simulink model "simulate_H_inf"  (R2013b)
settings: Solver=FixedStepDiscrete  StartTime=0.0  StopTime=100  FixedStep=T_s  RelTol=1e-3
values from neighbouring files (symbols this model uses):
  A = [0 0                                                1 0 ... (first row only)    [H_inf_state_feedback.m]    (also in Hinf_discrete_state_feedback_control (Dogan Onur ARISOY's conflicted copy 2017-02-06).m = a; Hinf_discrete_state_feedback_control.m = a; Hinf_discrete_state_feedback_control_ceyrek_tasit.m = a; bina_sistem.m = [zeros(4,4)         eye(4))
  B1 = [0;0;0;k2/m2]    [H_inf_state_feedback.m]    (also in Hinf_discrete_state_feedback_control (Dogan Onur ARISOY's conflicted copy 2017-02-06).m = b(:,1:size(Bc1,2)); Hinf_discrete_state_feedback_control.m = b(:,1:size(Bc1,2)); Hinf_discrete_state_feedback_control_ceyrek_tasit.m = b(:,1:size(Bc1,2)); bina_sistem.m = zeros(8,2))
  C = c(1:size(Cc1,1),:)    [Hinf_discrete_state_feedback_control (Dogan Onur ARISOY's conflicted copy 2017-02-06).m]    (also in Hinf_discrete_state_feedback_control.m; Hinf_discrete_state_feedback_control_ceyrek_tasit.m; bina_sistem.m = [c1+c2          -c2              0             0; dis_state_space.m)
  K = W*inv(X)    [H_inf_state_feedback.m]    (also in Hinf_discrete_state_feedback_control (Dogan Onur ARISOY's conflicted copy 2017-02-06).m = Y*Q^-1; Hinf_discrete_state_feedback_control.m = [k1 -k1;-k1 k1+k2]; Hinf_discrete_state_feedback_control_ceyrek_tasit.m = Y*Q^-1; LMI_state.m)
  T_s = 1e-6    (= 1e-06)    [Hinf_discrete_state_feedback_control (Dogan Onur ARISOY's conflicted copy 2017-02-06).m]    (also in Hinf_discrete_state_feedback_control.m = 0.0001; Hinf_discrete_state_feedback_control_ceyrek_tasit.m = 0.01; bench__lmi_state_hinf.m = 0.01; bina__lmi_state_hinf.m = 0.01)
settings Model: Creator=mert  LastModifiedBy=oguzhan
settings DebuggingCC: StateNameClashWarn=warning

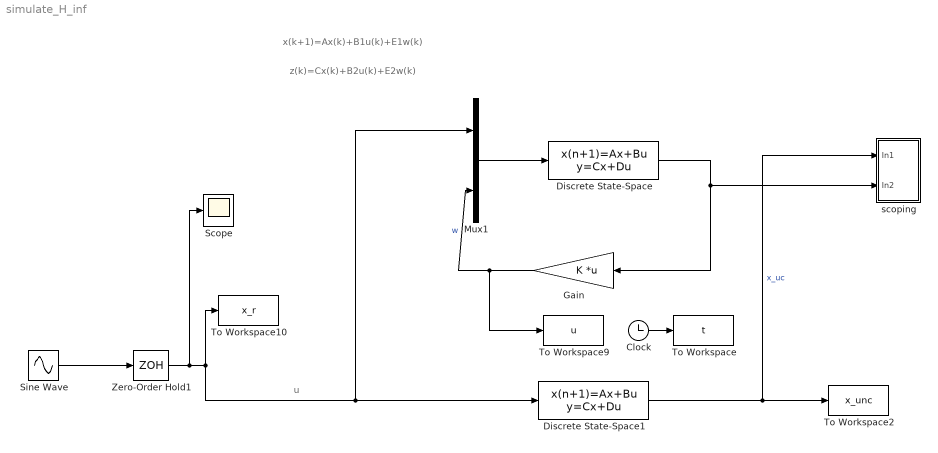
== system simulate_H_inf ==
  note: u
  note: z(k)=Cx(k)+B2u(k)+E2w(k)
  note: x(k+1)=Ax(k)+B1u(k)+E1w(k)
  Clock : Clock
  Discrete State-Space : DiscreteStateSpace  A=A  B=[B1 E1]  C=C  D=zeros(size(C,1),size([B1 E1],2))  SampleTime=T_s
  Discrete State-Space1 : DiscreteStateSpace  A=A  B=B1  C=C  D=zeros(size(C,1),size([B1],2))  SampleTime=T_s
  Gain : Gain  Gain=K  Multiplication=Matrix(K*u) (u vector)
  Mux1 : Mux  Inputs=2
  Scope : Scope
  Sine Wave : Sin  SampleTime=0
  To Workspace : ToWorkspace  VariableName=t  SampleTime=-1
  To Workspace10 : ToWorkspace  VariableName=x_r  SampleTime=-1
  To Workspace2 : ToWorkspace  VariableName=x_unc  SampleTime=-1  SaveFormat=Structure With Time
  To Workspace9 : ToWorkspace  VariableName=u  SampleTime=-1
  Zero-Order Hold1 : ZeroOrderHold  SampleTime=T_s
  scoping : Subsystem
  wires:
  Sine Wave/1 -> Zero-Order Hold1/1
  Clock/1 -> To Workspace/1
  Gain/1 -> Mux1/2, To Workspace9/1  "w"
  Mux1/1 -> Discrete State-Space/1
  Discrete State-Space1/1 -> scoping/1(In1), To Workspace2/1  "x_uc"
  Discrete State-Space/1 -> Gain/1, scoping/2(In2)
  Zero-Order Hold1/1 -> Scope/1, Mux1/1, Discrete State-Space1/1, To Workspace10/1

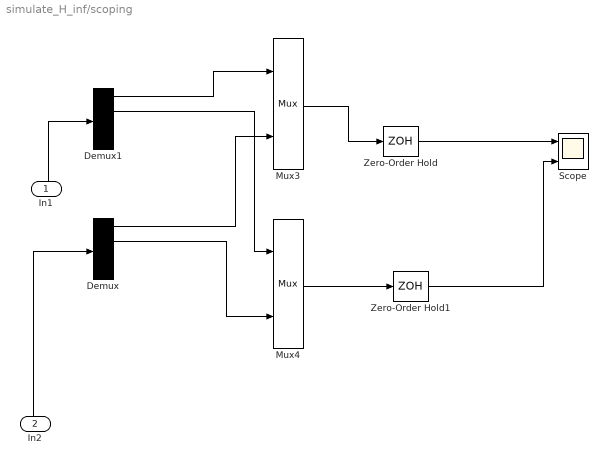
== system simulate_H_inf/scoping ==
  In1 : Inport
  In2 : Inport  Port=2
  Demux : Demux
  Demux1 : Demux
  Mux3 : Mux  Inputs=2
  Mux4 : Mux  Inputs=2
  Scope : Scope  NumInputPorts=2
      settings: TickLabels=on  ShowLegends=on  YMin=-5~-5  YMax=5~5  SampleTime=0.001
  Zero-Order Hold : ZeroOrderHold  SampleTime=0.001
  Zero-Order Hold1 : ZeroOrderHold  SampleTime=0.001
  wires:
  Mux4/1 -> Zero-Order Hold1/1
  Demux/1 -> Mux3/2
  Demux1/2 -> Mux4/1
  Mux3/1 -> Zero-Order Hold/1
  In1/1 -> Demux1/1
  In2/1 -> Demux/1
  Demux1/1 -> Mux3/1
  Demux/2 -> Mux4/2
  Zero-Order Hold/1 -> Scope/1
  Zero-Order Hold1/1 -> Scope/2
